simulink model "pendulum_crasilum"  (R2015a)
settings: Solver=ode45  StartTime=0.0  StopTime=10.0  RelTol=1e-3
libraries: vrlib x2
settings Model: Creator=Daniel  LastModifiedBy=Daniel

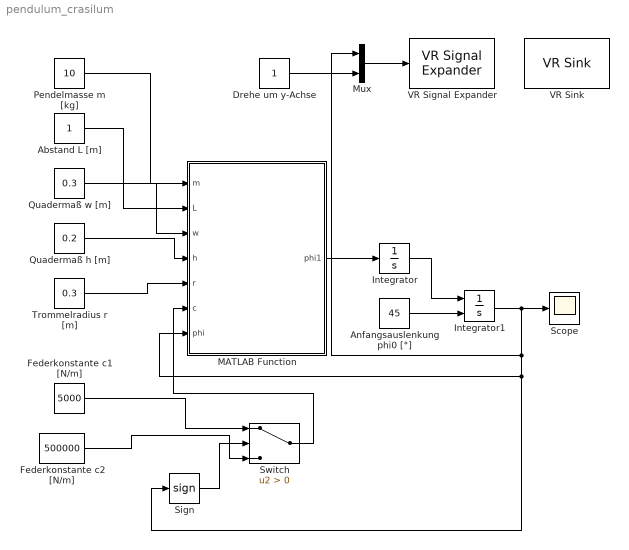
== system pendulum_crasilum ==
  Abstand L [m] : Constant
  Anfangsauslenkung phi0 [°] : Constant  Value=45
  Drehe um y-Achse : Constant
  Federkonstante c1 [N/m] : Constant  Value=5000
  Federkonstante c2 [N/m] : Constant  Value=500000
  Integrator : Integrator
  Integrator1 : Integrator  InitialConditionSource=external
  MATLAB Function : MATLAB Function  TreatAsAtomicUnit=on
  Mux : Mux  Inputs=2
  Pendelmasse m [kg] : Constant  Value=10
  Quadermaß h [m] : Constant  Value=0.2
  Quadermaß w [m] : Constant  Value=0.3
  Scope : Scope
  Sign : Signum
  Switch : Switch  Criteria=u2 > Threshold
  Trommelradius r [m] : Constant  Value=0.3
  VR Signal Expander : vrlib/VR Signal Expander  outwidth=4  outidx=[2 4]
  VR Sink : vrlib/VR Sink  InstantiateOnLoad=on  SampleTime=0.1  ViewEnable=on  RemoteChange=off  RemoteView=off  WorldFileName=alt\CrazyPendlm.wrl  AutoView=off  VideoDimensions=[]  AllowVariableSize=off
  wires:
  Pendelmasse m [kg]/1 -> MATLAB Function/1(m)
  Abstand L [m]/1 -> MATLAB Function/2(L)
  Quadermaß w [m]/1 -> MATLAB Function/3(w)
  Quadermaß h [m]/1 -> MATLAB Function/4(h)
  Trommelradius r [m]/1 -> MATLAB Function/5(r)
  Anfangsauslenkung phi0 [°]/1 -> Integrator1/2
  Switch/1 -> MATLAB Function/6(c)
  Federkonstante c1 [N/m]/1 -> Switch/1
  Federkonstante c2 [N/m]/1 -> Switch/3
  Sign/1 -> Switch/2
  MATLAB Function/1(phi1) -> Integrator/1
  Mux/1 -> VR Signal Expander/1
  Integrator/1 -> Integrator1/1
  Integrator1/1 -> Mux/1, MATLAB Function/7(phi), Sign/1, Scope/1
  Drehe um y-Achse/1 -> Mux/2

== matlab function pendulum_crasilum/MATLAB Function ==
  data: m input; L input; w input; h input; r input; c input; phi input; phi1 output
function phi1 = winkelbeschleunigung(m, L, w, h, r, c, phi)
    phiBog = phi0 * pi/180;
    u = (-c*2*pi*r^2*cos(phiBog)*(phi/360)) / ((1/12)*m*(w^2+h^2) + m*(L+(h/2))^2);
    phi = u; % winkelbeschleunigung
